simulink model "model_8"  (R2020a)
settings: Solver=VariableStepAuto  StartTime=0.0  StopTime=10.0  RelTol=1e-3
settings Model: Creator=Notnik_kg  LastModifiedBy=Notnik_kg

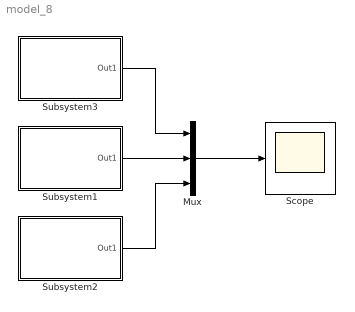
== system model_8 ==
  Mux : Mux  Inputs=3
  Scope : Scope
  Subsystem1 : Subsystem
  Subsystem2 : Subsystem
  Subsystem3 : Subsystem
  wires:
  Subsystem3/1(Out1) -> Mux/1
  Subsystem1/1(Out1) -> Mux/2
  Subsystem2/1(Out1) -> Mux/3
  Mux/1 -> Scope/1

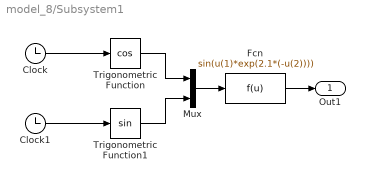
== system model_8/Subsystem1 ==
  Clock : Clock
  Clock1 : Clock
  Fcn : Fcn  Expr=sin(u(1)*exp(2.1*(-u(2))))
  Mux : Mux  Inputs=2
  Trigonometric Function : Trigonometry  Operator=cos
  Trigonometric Function1 : Trigonometry
  Out1 : Outport
  wires:
  Trigonometric Function/1 -> Mux/1
  Clock1/1 -> Trigonometric Function1/1
  Fcn/1 -> Out1/1
  Clock/1 -> Trigonometric Function/1
  Trigonometric Function1/1 -> Mux/2
  Mux/1 -> Fcn/1

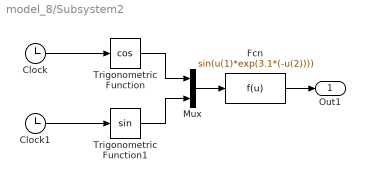
== system model_8/Subsystem2 ==
  Clock : Clock
  Clock1 : Clock
  Fcn : Fcn  Expr=sin(u(1)*exp(3.1*(-u(2))))
  Mux : Mux  Inputs=2
  Trigonometric Function : Trigonometry  Operator=cos
  Trigonometric Function1 : Trigonometry
  Out1 : Outport
  wires:
  Trigonometric Function/1 -> Mux/1
  Clock1/1 -> Trigonometric Function1/1
  Fcn/1 -> Out1/1
  Clock/1 -> Trigonometric Function/1
  Trigonometric Function1/1 -> Mux/2
  Mux/1 -> Fcn/1

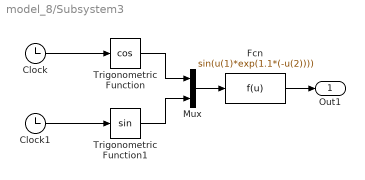
== system model_8/Subsystem3 ==
  Clock : Clock
  Clock1 : Clock
  Fcn : Fcn  Expr=sin(u(1)*exp(1.1*(-u(2))))
  Mux : Mux  Inputs=2
  Trigonometric Function : Trigonometry  Operator=cos
  Trigonometric Function1 : Trigonometry
  Out1 : Outport
  wires:
  Trigonometric Function/1 -> Mux/1
  Clock1/1 -> Trigonometric Function1/1
  Fcn/1 -> Out1/1
  Clock/1 -> Trigonometric Function/1
  Trigonometric Function1/1 -> Mux/2
  Mux/1 -> Fcn/1
